simulink model "mpcobj_1"  (R2023a)
settings: Solver=VariableStepAuto  StartTime=0.0  StopTime=20  RelTol=1e-3
libraries: mpclib x1, cstblocks x1
settings Model: Creator=xiong  LastModifiedBy=xiong

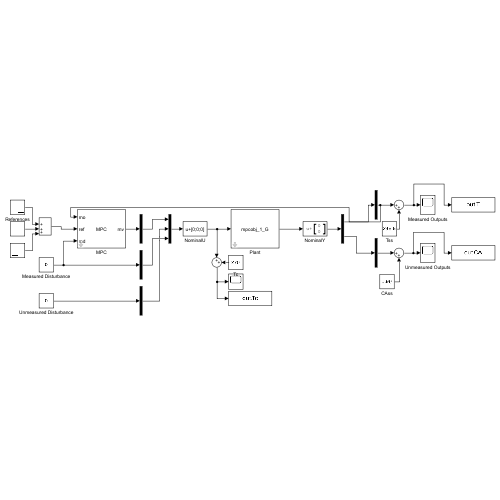
[thumbnail: Simulink's stored preview of the top-level diagram]
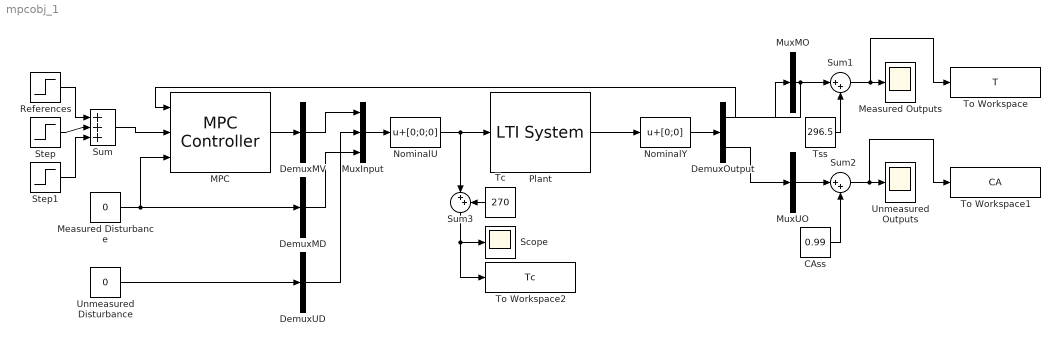
== system mpcobj_1 ==
  CAss : Constant  Value=0.99
  DemuxMD : Demux  Outputs=1
  DemuxMV : Demux  Outputs=1
  DemuxOutput : Demux  Outputs=2
  DemuxUD : Demux  Outputs=1
  MPC : mpclib/MPC Controller  SCDEnableBlockLinearizationSpecification=on  mpcobj=mpcobj_1_C  is_multiple=0  enable_value=0  return_u0=off  updateMPCinCallerWorkspace=on  md_inport=on  mv_inport=off  uref_inport=off  return_cost=off  return_mvseq=off  return_qpstatus=off  return_xseq=off  return_state=off  return_ovseq=off  state_inport=off  umin_inport=off  umax_inport=off  ymin_inport=off  ymax_inport=off  cc_inport=off  ywt_inport=off  uwt_inport=off  duwt_inport=off  rhoeps_inport=off  pm_inport=off  MaximumP=10  HorizonChoice=FixedHorizon  n_ts=0.1  n_p=15  n_mv=1  n_md=1  n_ud=1  n_mo=1  n_uo=1  BlockDataType=double  SampleTimeInherited=off  switch_inport=off
  Measured Disturbance : Constant  Value=0
  Measured Outputs : Scope
  MuxInput : Mux  Inputs=3
  MuxMO : Mux  Inputs=1
  MuxUO : Mux  Inputs=1
  NominalU : Bias  Bias=[0;0;0]
  NominalY : Bias  Bias=[0;0]
  Plant : cstblocks/LTI System  sys=mpcobj_1_G  IC=[]
  References : Step  Time=12  Before=[0;0]  After=[-40;0]  SampleTime=0.1
  Scope : Scope
  Step : Step  Time=8  Before=[0 0]  After=[20 0]  SampleTime=0.1
  Step1 : Step  Time=4  After=3.5  SampleTime=0.1
  Sum : Sum  Inputs=|+++
  Sum1 : Sum  Inputs=|++
  Sum2 : Sum  Inputs=|++
  Sum3 : Sum  Inputs=|++
  Tc : Constant  Value=270
  To Workspace : ToWorkspace  VariableName=T  SaveFormat=Timeseries  SampleTime=-1
  To Workspace1 : ToWorkspace  VariableName=CA  SaveFormat=Timeseries  SampleTime=-1
  To Workspace2 : ToWorkspace  VariableName=Tc  SaveFormat=Timeseries  SampleTime=-1
  Tss : Constant  Value=296.5
  Unmeasured Disturbance : Constant  Value=0
  Unmeasured Outputs : Scope
  wires:
  References/1 -> Sum/1
  Plant/1 -> NominalY/1
  NominalY/1 -> DemuxOutput/1
  MuxMO/1 -> Sum1/1, MPC/1
  MuxUO/1 -> Sum2/1
  DemuxOutput/1 -> MuxMO/1
  DemuxOutput/2 -> MuxUO/1
  MuxInput/1 -> NominalU/1
  NominalU/1 -> Sum3/1, Plant/1
  MPC/1 -> DemuxMV/1
  DemuxMV/1 -> MuxInput/1
  Measured Disturbance/1 -> MPC/3, DemuxMD/1
  DemuxMD/1 -> MuxInput/3
  Unmeasured Disturbance/1 -> DemuxUD/1
  DemuxUD/1 -> MuxInput/2
  Step/1 -> Sum/2
  Sum/1 -> MPC/2
  Tss/1 -> Sum1/2
  Sum1/1 -> To Workspace/1, Measured Outputs/1
  CAss/1 -> Sum2/2
  Sum2/1 -> To Workspace1/1, Unmeasured Outputs/1
  Sum3/1 -> To Workspace2/1, Scope/1
  Tc/1 -> Sum3/2
  Step1/1 -> Sum/3
